simulink model "OrbitPropagatorBlock"  (R2022a)
settings: Solver=FixedStepAuto  StartTime=0.0  StopTime=172800  FixedStep=60  MaxStep=60  MinStep=60  RelTol=1e-6  AbsTol=1e-7
model workspace (MATLAB code in the model file):
  | initialize6DOFSkyHogg;
settings Model: Creator=The MathWorks, Inc.  LastModifiedBy=Smit
settings SolverCC: MaxConsecutiveMinStep=5  AlgebraicLoopSolver=TrustRegion  AutoInsertRateTranBlk=on  InsertRTBMode=Never (minimum delay)  MinimalZcImpactIntegration=on
settings DataIOCC: SignalLogging=off  DSMLogging=off  SaveTime=off
settings OptimizationCC: EnhancedBackFolding=on  StrengthReduction=on  InitFltsAndDblsToZero=on  DifferentSizesBufferReuse=on
settings DebuggingCC: WriteAfterWriteMsg=DisableAll  AlgebraicLoopMsg=none  FcnCallInpInsideContextMsg=warning  UniqueDataStoreMsg=error  RootOutportRequireBusObject=none  StateNameClashWarn=warning  PregeneratedLibrarySubsystemCodeDiagnostic=none  StrictBusMsg=ErrorOnBusTreatedAsVector  SFUnexpectedBacktrackingDiag=warning  SFNoUnconditionalDefaultTransitionDiag=warning  SFExecutionAtInitializationDiag=none  SFMachineParentedDataDiag=warning  ArithmeticOperatorsInVariantConditions=warning
settings ModelReferenceCC: PropagateSignalLabelsOutOfModel=off
settings SFSimCC: SimUseLocalCustomCode=off
settings RTWCC: RTWUseLocalCustomCode=off  DLArmComputeVersion=19.05
settings CodeAppCC: StateflowObjectComments=on

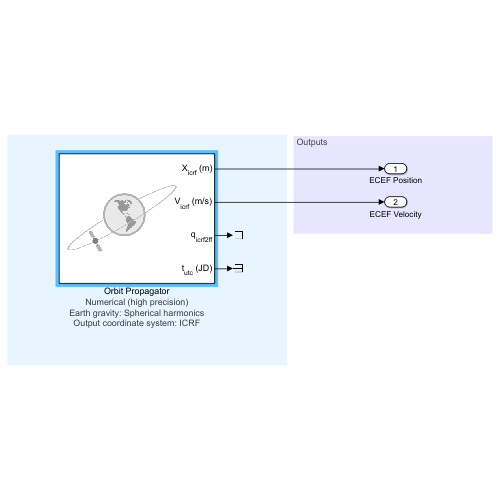
[thumbnail: Simulink's stored preview of the top-level diagram]
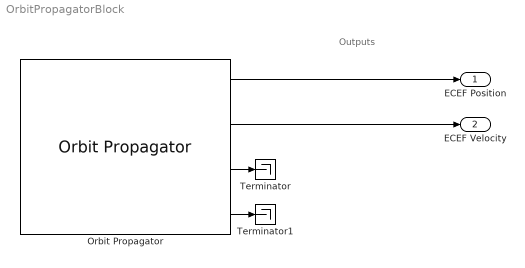
== system OrbitPropagatorBlock ==
  note: Outputs
  Orbit Propagator : OrbitPropagator  propagator=Numerical (high precision)  startDate=2458717.5  semiMajorAxis=mission.Satellite.SemiMajorAxis  eccentricity=mission.Satellite.Eccentricity  inclination=mission.Satellite.Inclination  raan=mission.Satellite.RAAN  argPeriapsis=mission.Satellite.ArgOfPeriapsis  trueAnomaly=mission.Satellite.TrueAnomaly  inertialPosition=[3649700.0 3308200.0 -4676600.0]  inertialVelocity=[-2750.8 6666.4 2573.4]  fixedPosition=[-4142689.0 -2676864.7 -4669861.6]  fixedVelocity=[1452.7 -6720.7 2568.1]  customR=3396200  customMu=4.305e13  customJ2=1.0826269e-03  customOmega=4.06125949e-3  outputTransform=on
      settings: AttributesFormatString=|
      | %<propagator>
      | Earth gravity: %<gravityModel>
      | Output coordinate system: %<outportFrame>
  Terminator : Terminator
  Terminator1 : Terminator
  ECEF Position : Outport
  ECEF Velocity : Outport  Port=2
  wires:
  Orbit Propagator/4 -> Terminator1/1
  Orbit Propagator/3 -> Terminator/1
  Orbit Propagator/1 -> ECEF Position/1
  Orbit Propagator/2 -> ECEF Velocity/1
